simulink model "nncontroller_5_50"  (R2021a)
(part 7 of 14)

  "IW{3,2}(50,:)'" : Constant  Value=[0.83646202146274173383488914623740129172801971435546875;0.977190867662071749322194591513834893703460693359375;0.70334945451090502555047123678377829492092132568359375;-0.499723725602324420069777488606632687151432037353515625;-0.286316455408377745772696698622894473373889923095703125;0.97778380580427681767474723528721369802951812744140625;0.5769785555966870926880574188544414937496185302734375;-0.50500217511694300842606253354460932314395904541015625;0.7621658406148894560061535230488516390323638916015625;-0.2560415054809486168352350432542152702808380126953125;-0.2174563075880605877987505891724140383303165435791015625;0.815660187555153459726398068596608936786651611328125;0.1513589200511942234328444101265631616115570068359375;0.95674695549343968803412963097798638045787811279296875;0.27261356752056276064877238241024315357208251953125;0.061257088775262591440196047187782824039459228515625;0.4606612352172587687704208292416296899318695068359375;0.649813191031489711946278475807048380374908447265625;-0.34187341806804472099656777572818100452423095703125;0.32114719342053599238084871103637851774692535400390625;-0.035206851792007665125083804014138877391815185546875;0.407108497673856872811626317343325354158878326416015625;0.8415826277085844964176430949009954929351806640625;-0.592589327713046731815893508610315620899200439453125;0.393217846957899297422045492567121982574462890625;0.820437120278952658480875470559112727642059326171875;-0.4840750214023754605108251780620776116847991943359375;0.63971487990579145588299070368520915508270263671875;-0.29878521510639577396517552188015542924404144287109375;-0.0645891909034566058522841558442451059818267822265625;0.5335980497254866339318368773092515766620635986328125;-0.454085039328891715282310315160430036485195159912109375;0.7375214448973197445269534000544808804988861083984375;-0.375397904462387022039848716303822584450244903564453125;-0.6629748397653560942899275687523186206817626953125;-0.80828198343561064032058993689133785665035247802734375;0.2945662639749688782586645174887962639331817626953125;0.98637982469137497343325549081782810389995574951171875;0.52994326971524607916563809340004809200763702392578125;-0.27073097164847104156848445200012065470218658447265625;0.1417750935767880804405649541877210140228271484375;0.488773933390067583104610093869268894195556640625;-0.081790040726720303343455498179537244141101837158203125;0.0392383240314788661606826281058602035045623779296875;0.7941249245912587184648145921528339385986328125;-0.446670707246191456274431175188510678708553314208984375;0.1575300533961102311675261944401427172124385833740234375;0.4345134853481216197224057395942509174346923828125;-0.368229314153628195516176901946892030537128448486328125;-0.1485648685626748954913267652955255471169948577880859375]
      mask Display: e = 0.06;c1 = [120 150 230]/255;c2 = ([120 150 230]+0)/383;c3 = ([120 150 230]+128)/383;patch([0 1 1 0],[0 0 1 1],c1);patch([0 1 1 1-e 1-e 0+e],[0 0 1 1-e 0+e 0+e],c2);patch([0 0 1 1-e 0+e 0+e],[0 1 1 1-e 1-e 0+e],c3);plot([0 1 1 0 0],[0 0 1 1 0]);disp('weights');
  "IW{3,2}(6,:)'" : Constant  Value=[-0.21089217855358466380266690975986421108245849609375;-0.944654393637833766916855893214233219623565673828125;-0.9916806460743803341983948484994471073150634765625;-0.5729987116772690125543476824532262980937957763671875;-0.686603870543795569147960122791118919849395751953125;-0.8033546357467005183394803680130280554294586181640625;-0.708979074004934428643309729523025453090667724609375;-0.613403429865451155222899615182541310787200927734375;0.71826333989041035721356820431537926197052001953125;0.8824577394499772964309158851392567157745361328125;-0.05593407269655603641922425595112144947052001953125;-0.344712587744194554062460156274028122425079345703125;-0.8651699259835561317544261328293941915035247802734375;0.4243620293664120968202269068569876253604888916015625;-0.50545896046434801718305607209913432598114013671875;-0.5385888279821118285184411433874629437923431396484375;0.5636452689061235421519313604221679270267486572265625;-0.8571934914055481247174839154467917978763580322265625;-0.2868626798432456492804476511082611978054046630859375;-0.9285204468279821821141695181722752749919891357421875;0.669521668021891169786385944462381303310394287109375;0.929797889836726287882129327044822275638580322265625;-0.5811298409768974604361346791847608983516693115234375;0.6505242199906258182551255231373943388462066650390625;0.68831217571675207267389851040206849575042724609375;-0.209063970115270780780747372773475944995880126953125;0.0954807265893926615518694234197027981281280517578125;-0.313662357571809824463571203523315489292144775390625;-0.1917599378655261421755540141020901501178741455078125;-0.8287971609069380019008121962542645633220672607421875;-0.3610905729112523498969267166103236377239227294921875;-0.75464091640410746464340263628400862216949462890625;0.2302649322276011378818338926066644489765167236328125;-0.603189941429487230806216757628135383129119873046875;-0.9080431327817006792457732444745488464832305908203125;-0.971109790362493452420267203706316649913787841796875;-0.467595391037224583641318531590513885021209716796875;0.0619856122954878241415599404717795550823211669921875;-0.1762920894775545921362436274648644030094146728515625;-0.36812532887225213329429607256315648555755615234375;-0.66823790467728994002527542761527001857757568359375;0.5944555973082543687269208021461963653564453125;0.8187868979933445867658292627311311662197113037109375;-0.5497687325267206492895866176695562899112701416015625;0.131729621078954028945418031071312725543975830078125;-0.212901590328389733741687450674362480640411376953125;0.6242380663177231614469064879813231527805328369140625;0.474326094530315600650283158756792545318603515625;-0.513524783536771334269133149064145982265472412109375;0.882715896881313799582358115003444254398345947265625]
      mask Display: e = 0.06;c1 = [120 150 230]/255;c2 = ([120 150 230]+0)/383;c3 = ([120 150 230]+128)/383;patch([0 1 1 0],[0 0 1 1],c1);patch([0 1 1 1-e 1-e 0+e],[0 0 1 1-e 0+e 0+e],c2);patch([0 0 1 1-e 0+e 0+e],[0 1 1 1-e 1-e 0+e],c3);plot([0 1 1 0 0],[0 0 1 1 0]);disp('weights');
  "IW{3,2}(7,:)'" : Constant  Value=[-0.7148834041469835920423747666063718497753143310546875;-0.595989075188219974421599545166827738285064697265625;-0.973089009262542159461872870451770722866058349609375;-0.253444704134684339891236959374509751796722412109375;0.747305043076913921851200939272530376911163330078125;-0.8169989021148207353206771585973910987377166748046875;-0.061309116331176749525866398471407592296600341796875;0.5337498551422885650907801391440443694591522216796875;0.4737549271315855126118776752264238893985748291015625;0.8717199464354603577476154896430671215057373046875;-0.867524008288675485545127230579964816570281982421875;-0.4780480191552511914920842173160053789615631103515625;-0.325216186264836171204706261050887405872344970703125;-0.7222055363876316302906843702658079564571380615234375;0.608448561159579792700924372184090316295623779296875;-0.140134297036857535800891128019429743289947509765625;-0.1257018015013369183208169488352723419666290283203125;-0.8518685799547383030727587538422085344791412353515625;0.61673196117660022963491428527049720287322998046875;0.4669848930259650199303678164142183959484100341796875;-0.4882197135327024373196991291479207575321197509765625;0.1554832991097521155410277060582302510738372802734375;0.03945978322943499705388603615574538707733154296875;-0.4992650203694222188488538449746556580066680908203125;-0.6930373288709759105330476813833229243755340576171875;-0.2054127664639768813259479429689235985279083251953125;0.8493874235362228741763601647107861936092376708984375;-0.4374535625036035657586808156338520348072052001953125;0.9811953352068181199996388386352919042110443115234375;-0.9803770622071514839745987046626396477222442626953125;0.332930424085648990484287423896603286266326904296875;-0.7704478771627798483478954949532635509967803955078125;-0.5044027164989544065321069865603931248188018798828125;-0.5009089952590810579380331546417437493801116943359375;-0.0385774541607606380466677364893257617950439453125;0.29189260406160233429773143143393099308013916015625;0.997773450812413198462991203996352851390838623046875;-0.622947820262125251389306868077255785465240478515625;-0.563687406587969785931591104599647223949432373046875;0.9828505483520058039204059241455979645252227783203125;0.5640463931695307575608921979437582194805145263671875;0.7201693078414328486047679689363576471805572509765625;-0.031597743121768662177828446147032082080841064453125;0.1612107960512856319468255605897866189479827880859375;-0.4839224207707715219584088117699138820171356201171875;0.817162808465457413120702767628245055675506591796875;-0.574048026350392870398309241863898932933807373046875;0.4510500961082948290226113385870121419429779052734375;0.734813408450053717757555205025710165500640869140625;0.0183691856730539004871616270975209772586822509765625]
      mask Display: e = 0.06;c1 = [120 150 230]/255;c2 = ([120 150 230]+0)/383;c3 = ([120 150 230]+128)/383;patch([0 1 1 0],[0 0 1 1],c1);patch([0 1 1 1-e 1-e 0+e],[0 0 1 1-e 0+e 0+e],c2);patch([0 0 1 1-e 0+e 0+e],[0 1 1 1-e 1-e 0+e],c3);plot([0 1 1 0 0],[0 0 1 1 0]);disp('weights');
  "IW{3,2}(8,:)'" : Constant  Value=[-0.6290643171196188543348171151592396199703216552734375;0.0927990440818173834003346200915984809398651123046875;-0.7832255656407227650817048925091512501239776611328125;-0.4799683432937544846907940154778771102428436279296875;-0.725738418220288394877570681273937225341796875;-0.628537623354552987819943155045621097087860107421875;-0.06653831742342486421648573013953864574432373046875;0.6712840302973563932908973583835177123546600341796875;0.8515654221873416584998039979836903512477874755859375;0.0016879792897828149733641112106852233409881591796875;0.5287081910740116796887377859093248844146728515625;0.5198561299639876676081939876894466578960418701171875;-0.512773450341348802083984992350451648235321044921875;0.239920415011121601622789967223070561885833740234375;0.926448267841846639925051931641064584255218505859375;0.8720339965520824687672529762494377791881561279296875;0.915779495911033247779187149717472493648529052734375;0.937751141832841472734116905485279858112335205078125;-0.5025043977412704254703612605226226150989532470703125;-0.6132896868834369907830250667757354676723480224609375;-0.927136293692168766966688053798861801624298095703125;-0.6956873128319909227457173983566462993621826171875;-0.688940326234318778375609326758421957492828369140625;0.935835046182273533332818260532803833484649658203125;0.5064617222498568605004720666329376399517059326171875;0.5893564065932912487966177650378085672855377197265625;-0.54737036235920744076111077447421848773956298828125;0.830311302890198721371461942908354103565216064453125;-0.06550595200353637181933663669042289257049560546875;-0.599655355699730829854843250359408557415008544921875;0.085790589581612675118549304897896945476531982421875;0.5233577530961071033743792213499546051025390625;0.7054488913645753367376300957403145730495452880859375;-0.838162394786963194093232232262380421161651611328125;-0.5411291141775420587833878016681410372257232666015625;0.4535156704367597768623454612679779529571533203125;0.826240140279271173540109884925186634063720703125;0.028297814163877443860428684274666011333465576171875;0.291859468192750881598840351216495037078857421875;0.2822718337718110870326881922665052115917205810546875;0.9068726141736049850550216433475725352764129638671875;0.498552416901822059713822454796172678470611572265625;0.4578126645211859635509199506486766040325164794921875;-0.4586949838971128290410206318483687937259674072265625;-0.20194176729794310887200481374748051166534423828125;0.0917169427402690917716654439573176205158233642578125;-0.660886177141787545252782365423627197742462158203125;0.261148537253188095519362832419574260711669921875;0.1408367470769114060402671384508721530437469482421875;-0.003727713761545903281557912123389542102813720703125]
      mask Display: e = 0.06;c1 = [120 150 230]/255;c2 = ([120 150 230]+0)/383;c3 = ([120 150 230]+128)/383;patch([0 1 1 0],[0 0 1 1],c1);patch([0 1 1 1-e 1-e 0+e],[0 0 1 1-e 0+e 0+e],c2);patch([0 0 1 1-e 0+e 0+e],[0 1 1 1-e 1-e 0+e],c3);plot([0 1 1 0 0],[0 0 1 1 0]);disp('weights');
  "IW{3,2}(9,:)'" : Constant  Value=[-0.7180109453942307151663726472179405391216278076171875;0.4208488203312790165711021472816355526447296142578125;-0.5124977590229919943709546714671887457370758056640625;-0.0875698046295754206624906146316789090633392333984375;0.083585183795706452514195916592143476009368896484375;0.1343947896103030448244908257038332521915435791015625;-0.1086558606387473258081399762886576354503631591796875;0.746755981481229458296411394258029758930206298828125;-0.780538514604703248522810099530033767223358154296875;-0.3478911741412928915195834633777849376201629638671875;-0.0201222642400182838429145704139955341815948486328125;-0.722887508353117436143975282902829349040985107421875;-0.9228409692260639562988444595248438417911529541015625;0.2774100021360677015280771229299716651439666748046875;0.1101055658239840084888783167116343975067138671875;-0.5909142336556201247077524385531432926654815673828125;-0.49278954184118095582789464970119297504425048828125;0.1404176242759664905435101900366134941577911376953125;0.1168990672529250929301269934512674808502197265625;-0.6555689810894909097527261110371910035610198974609375;0.7517134949877435357024069162434898316860198974609375;-0.5139580440746092104831177493906579911708831787109375;-0.614748739004576716382644008263014256954193115234375;0.8948836729938960399266534295747987926006317138671875;0.10068524456071603623286137008108198642730712890625;0.7226576111382196909715958099695853888988494873046875;0.405834158953896295685126460739411413669586181640625;-0.084512559572376577676777742453850805759429931640625;-0.02940661646818742980258321040309965610504150390625;-0.7160257116470993832280100832576863467693328857421875;0.441557553708751271415167138911783695220947265625;-0.5084050784912488296640731277875602245330810546875;0.9547788981548344100502845321898348629474639892578125;0.3735187148649163901836800505407154560089111328125;-0.054114836442081593048669674317352473735809326171875;-0.161942628656617682025853355298750102519989013671875;0.158217058560797152466648185509257018566131591796875;-0.3187846031292718151917142677120864391326904296875;-0.0185493090996315945773176281363703310489654541015625;-0.636899436930637108389419154264032840728759765625;-0.0486929044319348580671658055507577955722808837890625;-0.56330615388473592730633754399605095386505126953125;-0.2209116787154783434488081184099428355693817138671875;-0.0996371774297248880003508020308800041675567626953125;0.3335899811927747204975958084105513989925384521484375;-0.062654348408754945154441884369589388370513916015625;0.568799198791368088024000826408155262470245361328125;0.176755553002120091576898630592040717601776123046875;0.639411860199419646022533925133757293224334716796875;-0.393864521715036719484714922145940363407135009765625]
      mask Display: e = 0.06;c1 = [120 150 230]/255;c2 = ([120 150 230]+0)/383;c3 = ([120 150 230]+128)/383;patch([0 1 1 0],[0 0 1 1],c1);patch([0 1 1 1-e 1-e 0+e],[0 0 1 1-e 0+e 0+e],c2);patch([0 0 1 1-e 0+e 0+e],[0 1 1 1-e 1-e 0+e],c3);plot([0 1 1 0 0],[0 0 1 1 0]);disp('weights');
  Mux : Mux  Inputs=50
      mask Display: e = 0.06;c1 = [120 150 230]/255;c2 = ([120 150 230]+0)/383;c3 = ([120 150 230]+128)/383;patch([0 1 1 0],[0 0 1 1],c1);patch([0 1 1 1-e 1-e 0+e],[0 0 1 1-e 0+e 0+e],c2);patch([0 0 1 1-e 0+e 0+e],[0 1 1 1-e 1-e 0+e],c3);plot([0 1 1 0 0],[0 0 1 1 0]);disp('Mux');
  dotprod{1..50} (50 alike) : neural/Weight Functions/dotprod
  "lz{3,2}" : Outport
      mask Display: e = 0.06;c1 = [120 230 180]/255;c2 = ([120 230 180]+0)/(256+128);c3 = ([120 230 180]+128)/(256+128);patch([0 1 1 0],[0 0 1 1],c1);patch([0 1 1 1-e 1-e 0+e],[0 0 1 1-e 0+e 0+e],c2);patch([0 0 1 1-e 0+e 0+e],[0 1 1 1-e 1-e 0+e],c3);plot([0 1 1 0 0],[0 0 1 1 0]);
  wires:
  "IW{3,2}(1,:)'"/1 -> dotprod1/1
  "ad{3,2}"/1 -> dotprod1/2, dotprod2/2, dotprod3/2, dotprod4/2, dotprod5/2, dotprod6/2, dotprod7/2, dotprod8/2, dotprod9/2, dotprod10/2, dotprod11/2, dotprod12/2, dotprod13/2, dotprod14/2, dotprod15/2, dotprod16/2, dotprod17/2, dotprod18/2, dotprod19/2, dotprod20/2, dotprod21/2, dotprod22/2, dotprod23/2, dotprod24/2, dotprod25/2, dotprod26/2, dotprod27/2, dotprod28/2, dotprod29/2, dotprod30/2, dotprod31/2, dotprod32/2, dotprod33/2, dotprod34/2, dotprod35/2, dotprod36/2, dotprod37/2, dotprod38/2, dotprod39/2, dotprod40/2, dotprod41/2, dotprod42/2, dotprod43/2, dotprod44/2, dotprod45/2, dotprod46/2, dotprod47/2, dotprod48/2, dotprod49/2, dotprod50/2
  dotprod1/1 -> Mux/1
  "IW{3,2}(2,:)'"/1 -> dotprod2/1
  dotprod2/1 -> Mux/2
  "IW{3,2}(3,:)'"/1 -> dotprod3/1
  dotprod3/1 -> Mux/3
  "IW{3,2}(4,:)'"/1 -> dotprod4/1
  dotprod4/1 -> Mux/4
  "IW{3,2}(5,:)'"/1 -> dotprod5/1
  dotprod5/1 -> Mux/5
  "IW{3,2}(6,:)'"/1 -> dotprod6/1
  dotprod6/1 -> Mux/6
  "IW{3,2}(7,:)'"/1 -> dotprod7/1
  dotprod7/1 -> Mux/7
  "IW{3,2}(8,:)'"/1 -> dotprod8/1
  dotprod8/1 -> Mux/8
  "IW{3,2}(9,:)'"/1 -> dotprod9/1
  dotprod9/1 -> Mux/9
  "IW{3,2}(10,:)'"/1 -> dotprod10/1
  dotprod10/1 -> Mux/10
  "IW{3,2}(11,:)'"/1 -> dotprod11/1
  dotprod11/1 -> Mux/11
  "IW{3,2}(12,:)'"/1 -> dotprod12/1
  dotprod12/1 -> Mux/12
  "IW{3,2}(13,:)'"/1 -> dotprod13/1
  dotprod13/1 -> Mux/13
  "IW{3,2}(14,:)'"/1 -> dotprod14/1
  dotprod14/1 -> Mux/14
  "IW{3,2}(15,:)'"/1 -> dotprod15/1
  dotprod15/1 -> Mux/15
  "IW{3,2}(16,:)'"/1 -> dotprod16/1
  dotprod16/1 -> Mux/16
  "IW{3,2}(17,:)'"/1 -> dotprod17/1
  dotprod17/1 -> Mux/17
  "IW{3,2}(18,:)'"/1 -> dotprod18/1
  dotprod18/1 -> Mux/18
  "IW{3,2}(19,:)'"/1 -> dotprod19/1
  dotprod19/1 -> Mux/19
  "IW{3,2}(20,:)'"/1 -> dotprod20/1
  dotprod20/1 -> Mux/20
  "IW{3,2}(21,:)'"/1 -> dotprod21/1
  dotprod21/1 -> Mux/21
  "IW{3,2}(22,:)'"/1 -> dotprod22/1
  dotprod22/1 -> Mux/22
  "IW{3,2}(23,:)'"/1 -> dotprod23/1
  dotprod23/1 -> Mux/23
  "IW{3,2}(24,:)'"/1 -> dotprod24/1
  dotprod24/1 -> Mux/24
  "IW{3,2}(25,:)'"/1 -> dotprod25/1
  dotprod25/1 -> Mux/25
  "IW{3,2}(26,:)'"/1 -> dotprod26/1
  dotprod26/1 -> Mux/26
  "IW{3,2}(27,:)'"/1 -> dotprod27/1
  dotprod27/1 -> Mux/27
  "IW{3,2}(28,:)'"/1 -> dotprod28/1
  dotprod28/1 -> Mux/28
  "IW{3,2}(29,:)'"/1 -> dotprod29/1
  dotprod29/1 -> Mux/29
  "IW{3,2}(30,:)'"/1 -> dotprod30/1
  dotprod30/1 -> Mux/30
  "IW{3,2}(31,:)'"/1 -> dotprod31/1
  dotprod31/1 -> Mux/31
  "IW{3,2}(32,:)'"/1 -> dotprod32/1
  dotprod32/1 -> Mux/32
  "IW{3,2}(33,:)'"/1 -> dotprod33/1
  dotprod33/1 -> Mux/33
  "IW{3,2}(34,:)'"/1 -> dotprod34/1
  dotprod34/1 -> Mux/34
  "IW{3,2}(35,:)'"/1 -> dotprod35/1
  dotprod35/1 -> Mux/35
  "IW{3,2}(36,:)'"/1 -> dotprod36/1
  dotprod36/1 -> Mux/36
  "IW{3,2}(37,:)'"/1 -> dotprod37/1
  dotprod37/1 -> Mux/37
  "IW{3,2}(38,:)'"/1 -> dotprod38/1
  dotprod38/1 -> Mux/38
  "IW{3,2}(39,:)'"/1 -> dotprod39/1
  dotprod39/1 -> Mux/39
  "IW{3,2}(40,:)'"/1 -> dotprod40/1
  dotprod40/1 -> Mux/40
  "IW{3,2}(41,:)'"/1 -> dotprod41/1
  dotprod41/1 -> Mux/41
  "IW{3,2}(42,:)'"/1 -> dotprod42/1
  dotprod42/1 -> Mux/42
  "IW{3,2}(43,:)'"/1 -> dotprod43/1
  dotprod43/1 -> Mux/43
  "IW{3,2}(44,:)'"/1 -> dotprod44/1
  dotprod44/1 -> Mux/44
  "IW{3,2}(45,:)'"/1 -> dotprod45/1
  dotprod45/1 -> Mux/45
  "IW{3,2}(46,:)'"/1 -> dotprod46/1
  dotprod46/1 -> Mux/46
  "IW{3,2}(47,:)'"/1 -> dotprod47/1
  dotprod47/1 -> Mux/47
  "IW{3,2}(48,:)'"/1 -> dotprod48/1
  dotprod48/1 -> Mux/48
  "IW{3,2}(49,:)'"/1 -> dotprod49/1
  dotprod49/1 -> Mux/49
  "IW{3,2}(50,:)'"/1 -> dotprod50/1
  dotprod50/1 -> Mux/50
  Mux/1 -> "lz{3,2}"/1
